simulink model "MPEG_Decoder"  (R2020b)
settings: Solver=VariableStepDiscrete  StartTime=0.0  StopTime=stopTime  RelTol=1e-3
values from neighbouring files (symbols this model uses):
  n = [1:C]    [pdfMM1K.m]
  period = 1/fps    (= 0.0166666666667)    [server_report.m]
undefined symbols (not defined in the file or in its folder): m
settings Model: Creator=Ander  LastModifiedBy=Ander
settings SolverCC: ZeroCrossControl=DisableAll

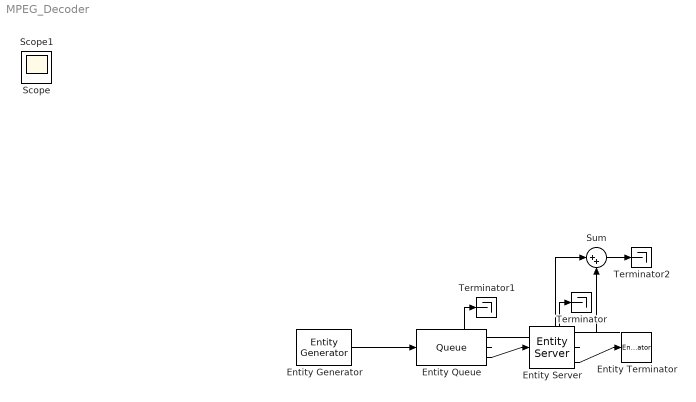
== system MPEG_Decoder ==
  Entity Generator : EntityGenerator  OutputPortMessageModes=m  Period=period  GenerateEntityAtSimulationStart=off  GenerateAction=|  AttributeName=Node|Size  AttributeInitialValue=1|0.02  EntityType=Structured  EntityTypeName=Entity
      | persistent rngInit;
      | if isempty(rngInit)
      |     seed = mySeed;
      |     rng(seed);
      |     rngInit = true;
      | end
      | V = [1 2 3 4];
      | S = [0.02 0.015 0.01 0.005];
      | P = [ 0.01 0.40 0.19 0.40;
      |       0.15 0.80 0.05 0.00;
      |       0.03 0.25 0.70 0.02;
      |       0.40 0.00 0.10 0.50 ];
      | 
      | persistent currentNode
      | if isempty(currentNode)
      |     currentNode = 1;
      | end
      | 
      | entity.Node = currentNode;
      | entity.Size = S(currentNode);
      | 
      | switch currentNode
      |     case 1
      |         currentNode = randsample(V, 1, true, P(1,:));
      |     case 2
      |         currentNode = randsample(V, 1, true, P(2,:));
      |     case 3
      |         currentNode = randsample(V, 1, true, P(3,:));
      |     otherwise
      |         currentNode = randsample(V, 1, true, P(4,:));
      | end
  Entity Queue : Queue  InputPortMessageModes=m  OutputPortMessageModes=n,n,m  Capacity=inf  NumberEntitiesInBlock=on  AverageWait=on
      settings: OutputPortMap=o1,o2,o5
  Entity Server : EntityServer  InputPortMessageModes=m  OutputPortMessageModes=n,n,m  Capacity=1  ServiceTimeSource=Attribute  ServiceTimeAttributeName=Size  NumberEntitiesInBlock=on  AverageWait=on
      settings: OutputPortMap=o1,o4,o9
  Entity Terminator : EntityTerminator  InputPortMessageModes=m
  Sum : Sum  Inputs=|++
  Terminator : Terminator
  Terminator1 : Terminator
  Terminator2 : Terminator
  Scope : Scope
  Scope1 : Scope
  wires:
  Entity Generator/1 -> Entity Queue/1
  Entity Queue/3 -> Entity Server/1
  Entity Server/3 -> Entity Terminator/1
  Entity Queue/2 -> Terminator1/1
  Entity Server/1 -> Sum/2
  Entity Queue/1 -> Sum/1
  Entity Server/2 -> Terminator/1
  Sum/1 -> Terminator2/1
